simulink model "smth"  (R2022b)
settings: Solver=VariableStepAuto  StartTime=0.0  StopTime=2.0  RelTol=1e-3
values from neighbouring files (symbols this model uses):
  k = K(i)    [UI.m]
  Tm = TM(i)    [UI.m]
  U_pr = Uall(i)    [UI.m]
settings Model: Creator=tameembourgi  LastModifiedBy=Alena

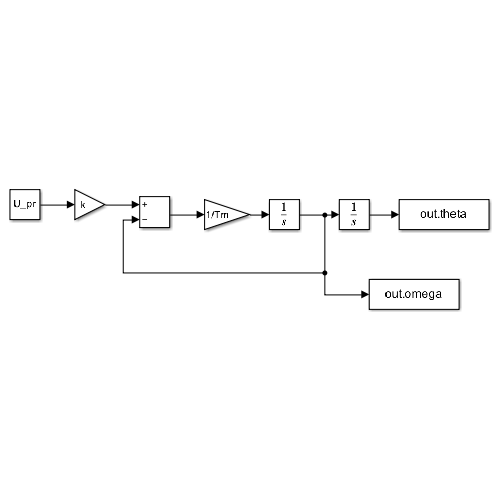
[thumbnail: Simulink's stored preview of the top-level diagram]
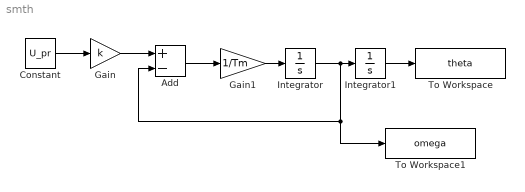
== system smth ==
  Add : Sum  Inputs=+-
  Constant : Constant  Value=U_pr
  Gain : Gain  Gain=k
  Gain1 : Gain  Gain=1/Tm
  Integrator : Integrator
  Integrator1 : Integrator
  To Workspace : ToWorkspace  VariableName=theta  SaveFormat=Timeseries  SampleTime=-1
  To Workspace1 : ToWorkspace  VariableName=omega  SaveFormat=Timeseries  SampleTime=-1
  wires:
  Constant/1 -> Gain/1
  Gain/1 -> Add/1
  Add/1 -> Gain1/1
  Gain1/1 -> Integrator/1
  Integrator/1 -> Add/2, To Workspace1/1, Integrator1/1
  Integrator1/1 -> To Workspace/1
